simulink model "enginetable"  (Simulink 6.0)
settings: Solver=FixedStepDiscrete  StartTime=0.0  StopTime=inf  FixedStep=1  RelTol=1e-3
PreLoadFcn:
  | load vedata
values from neighbouring files (symbols this model uses):
  X = [10 20 30 40 50 60 70 80 90 100]    [vedata.mat]
  Y = [0 200 400 600 800 1000 1200 1400 1600 1800 2000 2200 ... (36 elements, 36x1)]    [vedata.mat]
undefined symbols (not defined in the file or in its folder): plotmesh
libraries: simulink x3, spelookup x1
settings Model: Creator=beryilma  LastModifiedBy=rlandy
settings DataIOCC: SaveOutput=off  SaveTime=off  SignalLoggingName=sigsOut
settings OptimizationCC: BooleanDataType=off
settings DebuggingCC: CheckExecutionContextPreStartOutputMsg=on  CheckExecutionContextRuntimeOutputMsg=on  SolverPrmCheckMsg=none
settings HardwareCC: TargetUnknown=on
settings ModelReferenceCC: UpdateModelReferenceTargets=IfOutOfDate
settings GRTTargetCC: LifeSpan=inf
settings SFSimCC: SFSimApplyToAllLibs=on  SFSimBuildMode=Incremental

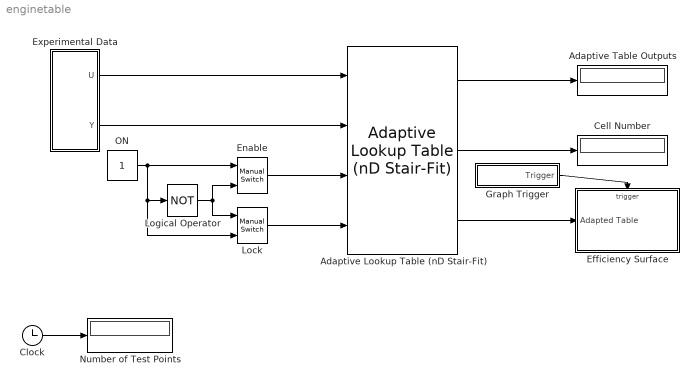
== system enginetable ==
  Adaptive Lookup Table (nD Stair-Fit) : spelookup/Adaptive Lookup Table (nD Stair-Fit)  Tb_NumDim=2  Bp_Cell={[X; 110], [Y; 7200]}  Tb_Input=off  Tb_Data=rand(10,36)  Tb_NumData=reshape(1:360,10,36)  Ad_Method=Sample mean (with forgetting)  Ad_Factor=0.98  Tb_Output=on  Ad_Enable=on  Ad_Lock=on  Ad_Range=Ignore
  Adaptive Table Outputs : Display
  Cell Number : Display
  Clock : Clock
      settings: Decimation=10
  Efficiency Surface : Subsystem  TreatAsAtomicUnit=on  EnableExecutionContextPropagation=on
  Enable : simulink/Signal Routing/Manual Switch  sw=1  action=0
  Experimental Data : Subsystem  EnableExecutionContextPropagation=on
  Graph Trigger : Subsystem  EnableExecutionContextPropagation=on
  Lock : simulink/Signal Routing/Manual Switch  sw=1  action=0
  Logical Operator : Logic  Operator=NOT
  Number of Test Points : Display
  ON : Constant
  wires:
  Experimental Data/1(U) -> Adaptive Lookup Table (nD Stair-Fit)/1
  Experimental Data/2(Y) -> Adaptive Lookup Table (nD Stair-Fit)/2
  Adaptive Lookup Table (nD Stair-Fit)/1 -> Adaptive Table Outputs/1
  Adaptive Lookup Table (nD Stair-Fit)/2 -> Cell Number/1
  Graph Trigger/1(Trigger) -> Efficiency Surface/Trigger
  Adaptive Lookup Table (nD Stair-Fit)/3 -> Efficiency Surface/1(Adapted Table)
  ON/1 -> Enable/1, Lock/2, Logical Operator/1
  Logical Operator/1 -> Lock/1, Enable/2
  Enable/1 -> Adaptive Lookup Table (nD Stair-Fit)/3
  Lock/1 -> Adaptive Lookup Table (nD Stair-Fit)/4
  Clock/1 -> Number of Test Points/1

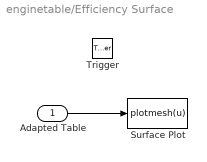
== system enginetable/Efficiency Surface ==
  Adapted Table : Inport  LatchInput=off
  Trigger : TriggerPort  ZeroCross=off
  Surface Plot : MATLABFcn  MATLABFcn=plotmesh(u)  OutputDimensions=0  Output1D=off
  wires:
  Adapted Table/1 -> Surface Plot/1

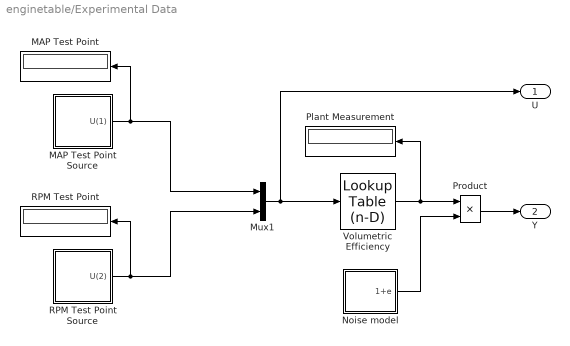
== system enginetable/Experimental Data ==
  MAP Test Point : Display
  MAP Test Point Source : Subsystem  EnableExecutionContextPropagation=on
  Mux1 : Mux  Inputs=2
  Noise model : Subsystem  EnableExecutionContextPropagation=on
  Plant Measurement : Display
  Product : Product  SaturateOnIntegerOverflow=on  InputSameDT=on
  RPM Test Point : Display
  RPM Test Point Source : Subsystem  EnableExecutionContextPropagation=on
  Volumetric Efficiency : simulink/Lookup Tables/Lookup Table (n-D)  numDimsPopupSelect=2  bp1=X  bp2=Y  bp3=[1:3]  bp4=[1:3]  bpcell={ [1:3], [1:3] }  explicitNumDims=2  searchMode=Binary Search  cacheBpFlag=off  vectorInputFlag=on  tableData=Z  interpMethod=Linear  extrapMethod=Linear  rangeErrorMode=None
  U : Outport
  Y : Outport  Port=2
  wires:
  Volumetric Efficiency/1 -> Plant Measurement/1, Product/1
  Mux1/1 -> U/1, Volumetric Efficiency/1
  RPM Test Point Source/1(U(2)) -> Mux1/2, RPM Test Point/1
  MAP Test Point Source/1(U(1)) -> Mux1/1, MAP Test Point/1
  Noise model/1(1+e) -> Product/2
  Product/1 -> Y/1

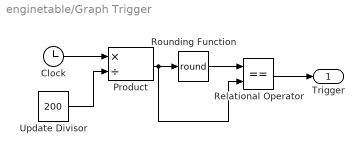
== system enginetable/Graph Trigger ==
  Clock : Clock
      settings: Decimation=10
  Product : Product  Inputs=*/  SaturateOnIntegerOverflow=on  InputSameDT=on
  Relational Operator : RelationalOperator  Operator===  ZeroCross=off  InputSameDT=on
  Rounding Function : Rounding  Operator=round
  Update Divisor : Constant  Value=200
  Trigger : Outport
  wires:
  Clock/1 -> Product/1
  Update Divisor/1 -> Product/2
  Product/1 -> Rounding Function/1, Relational Operator/2
  Rounding Function/1 -> Relational Operator/1
  Relational Operator/1 -> Trigger/1

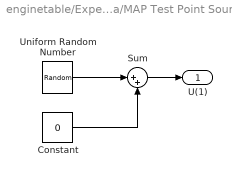
== system enginetable/Experimental Data/MAP Test Point Source ==
  Constant : Constant  Value=0
  Sum : Sum  Inputs=|++  SaturateOnIntegerOverflow=on  InputSameDT=on
  Uniform Random Number : UniformRandomNumber  Minimum=min(X) - 10  Maximum=max(X) + 10  Seed=3  SampleTime=0
  U(1) : Outport
  wires:
  Uniform Random Number/1 -> Sum/1
  Constant/1 -> Sum/2
  Sum/1 -> U(1)/1

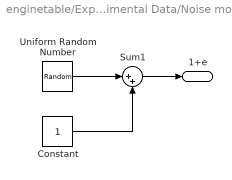
== system enginetable/Experimental Data/Noise model ==
  Constant : Constant
  Sum1 : Sum  Inputs=|++  SaturateOnIntegerOverflow=on  InputSameDT=on
  Uniform Random Number : UniformRandomNumber  Minimum=-0.05  Maximum=+0.05  Seed=2  SampleTime=0
  1+e : Outport
  wires:
  Uniform Random Number/1 -> Sum1/1
  Constant/1 -> Sum1/2
  Sum1/1 -> 1+e/1

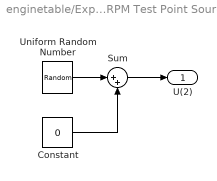
== system enginetable/Experimental Data/RPM Test Point Source ==
  Constant : Constant  Value=0
  Sum : Sum  Inputs=|++  SaturateOnIntegerOverflow=on  InputSameDT=on
  Uniform Random Number : UniformRandomNumber  Minimum=min(Y) - 100  Maximum=max(Y) + 100  SampleTime=0
  U(2) : Outport
  wires:
  Constant/1 -> Sum/2
  Uniform Random Number/1 -> Sum/1
  Sum/1 -> U(2)/1
